simulink model "simulation"  (R2022b)
settings: Solver=VariableStepAuto  StartTime=0.0  StopTime=3  RelTol=1e-3
values from neighbouring files (symbols this model uses):
  A = [0 1;10 0]    [LQRINIT.m]
  B = [0 -1]'    [LQRINIT.m]
  C = [1 0]    [LQRINIT.m]
  D = 0    [LQRINIT.m]
  K0 = lqr(A,B,Q0,R0)    [LQRINIT.m]
  K1 = lqr(A,B,Q1,R1)    [LQRINIT.m]
  K2 = lqr(A,B,Q2,R2)    [LQRINIT.m]
undefined symbols (not defined in the file or in its folder): Continuous, Time
libraries: ctrlSharedLib x3
settings Model: Creator=lenovo  LastModifiedBy=lenovo

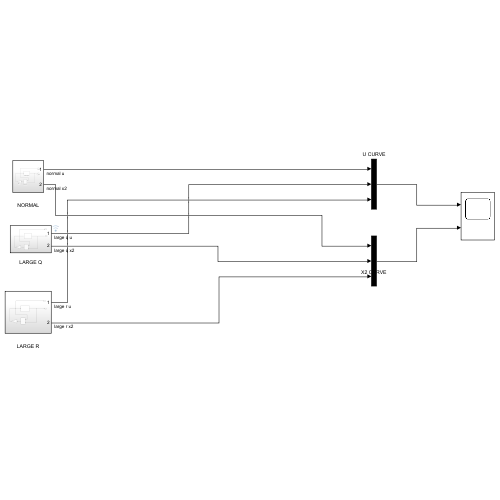
[thumbnail: Simulink's stored preview of the top-level diagram]
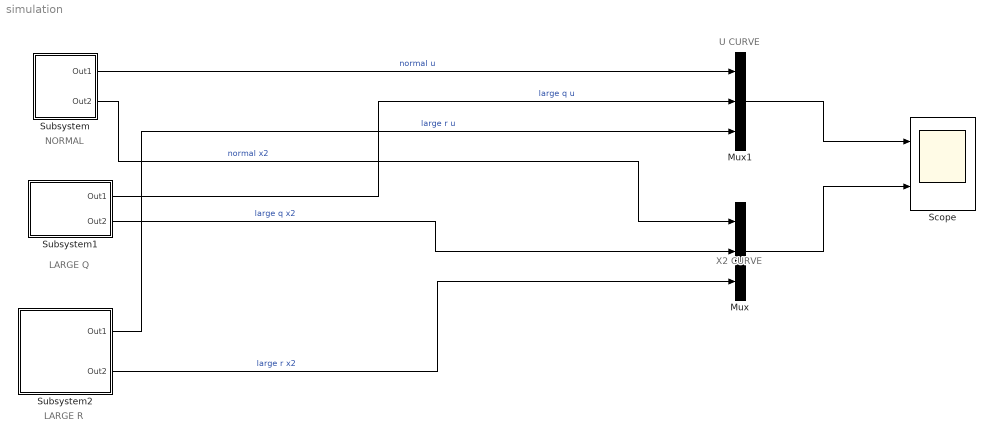
== system simulation ==
  note: LARGE R
  note: LARGE Q
  note: NORMAL
  note: U CURVE
  note: X2 CURVE
  Mux : Mux  Inputs=3
  Mux1 : Mux  Inputs=3
  Scope : Scope  NumInputPorts=2
  Subsystem : Subsystem
  Subsystem1 : Subsystem
  Subsystem2 : Subsystem
  wires:
  Subsystem/1(Out1) -> Mux1/1  "normal u"
  Subsystem/2(Out2) -> Mux/1  "normal x2"
  Subsystem2/2(Out2) -> Mux/3  "large r x2"
  Subsystem1/2(Out2) -> Mux/2  "large q x2"
  Subsystem1/1(Out1) -> Mux1/2  "large q u"
  Subsystem2/1(Out1) -> Mux1/3  "large r u"
  Mux1/1 -> Scope/1
  Mux/1 -> Scope/2

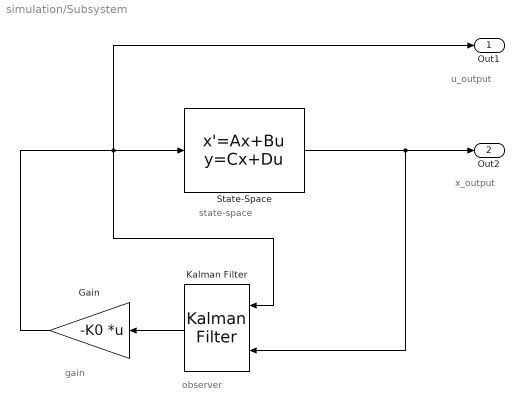
== system simulation/Subsystem ==
  note: state-space
  note: observer
  note: gain
  note: x_output
  note: u_output
  Gain : Gain  Gain=-K0  Multiplication=Matrix(K*u)
  Kalman Filter : ctrlSharedLib/Kalman Filter  TimeDomain=Continuous-Time  UseCurrentEstimator=on  ModelSource=Individual A, B, C, D matrices  ModelSourceVariable=ss(0.95,1,1,0,1)  A=A  B=B  C=C  D=D  NumberOfStates=1  NumberOfInputs=1  NumberOfOutputs=1  InitialEstimateSource=Dialog  X0=0  P0=10  UseK=off  UseGH=off  NumberOfProcessNoiseInputs=1  G=1  TimeInvariantG=on  H=0  TimeInvariantH=on  Q=0.05  TimeInvariantQ=on  R=1  TimeInvariantR=on  N=0  TimeInvariantN=on  AddInputPort=on  AddEnablePort=off  OutputEstimatedY=off  OutputP=off  Ts=-1
  State-Space : StateSpace  A=A  B=B  C=C  D=D  InitialCondition=5
  Out1 : Outport
  Out2 : Outport  Port=2
  wires:
  State-Space/1 -> Out2/1, Kalman Filter/2
  Gain/1 -> Kalman Filter/1, Out1/1, State-Space/1
  Kalman Filter/1 -> Gain/1

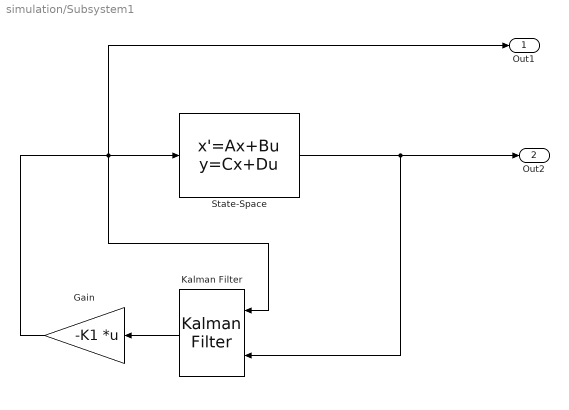
== system simulation/Subsystem1 ==
  Gain : Gain  Gain=-K1  Multiplication=Matrix(K*u)
  Kalman Filter : ctrlSharedLib/Kalman Filter  TimeDomain=Continuous-Time  UseCurrentEstimator=on  ModelSource=Individual A, B, C, D matrices  ModelSourceVariable=ss(0.95,1,1,0,1)  A=A  B=B  C=C  D=D  NumberOfStates=1  NumberOfInputs=1  NumberOfOutputs=1  InitialEstimateSource=Dialog  X0=0  P0=10  UseK=off  UseGH=off  NumberOfProcessNoiseInputs=1  G=1  TimeInvariantG=on  H=0  TimeInvariantH=on  Q=0.05  TimeInvariantQ=on  R=1  TimeInvariantR=on  N=0  TimeInvariantN=on  AddInputPort=on  AddEnablePort=off  OutputEstimatedY=off  OutputP=off  Ts=-1
  State-Space : StateSpace  A=A  B=B  C=C  D=D  InitialCondition=5
  Out1 : Outport
  Out2 : Outport  Port=2
  wires:
  State-Space/1 -> Out2/1, Kalman Filter/2
  Gain/1 -> Kalman Filter/1, Out1/1, State-Space/1
  Kalman Filter/1 -> Gain/1

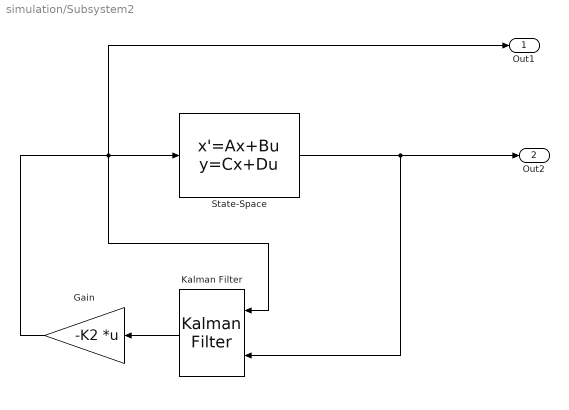
== system simulation/Subsystem2 ==
  Gain : Gain  Gain=-K2  Multiplication=Matrix(K*u)
  Kalman Filter : ctrlSharedLib/Kalman Filter  TimeDomain=Continuous-Time  UseCurrentEstimator=on  ModelSource=Individual A, B, C, D matrices  ModelSourceVariable=ss(0.95,1,1,0,1)  A=A  B=B  C=C  D=D  NumberOfStates=1  NumberOfInputs=1  NumberOfOutputs=1  InitialEstimateSource=Dialog  X0=0  P0=10  UseK=off  UseGH=off  NumberOfProcessNoiseInputs=1  G=1  TimeInvariantG=on  H=0  TimeInvariantH=on  Q=0.05  TimeInvariantQ=on  R=1  TimeInvariantR=on  N=0  TimeInvariantN=on  AddInputPort=on  AddEnablePort=off  OutputEstimatedY=off  OutputP=off  Ts=-1
  State-Space : StateSpace  A=A  B=B  C=C  D=D  InitialCondition=5
  Out1 : Outport
  Out2 : Outport  Port=2
  wires:
  State-Space/1 -> Out2/1, Kalman Filter/2
  Gain/1 -> Kalman Filter/1, Out1/1, State-Space/1
  Kalman Filter/1 -> Gain/1
